simulink model "xplane2matlab"  (R2016a)
settings: Solver=ode45  StartTime=0.0  StopTime=inf  RelTol=1e-3
libraries: xpcutilitieslib x2, xpcobsoletelib x2, instrumentlib x2
settings Model: Creator=IEE12  LastModifiedBy=Marcelo
settings DataIOCC: LimitDataPoints=on  SaveFormat=Array
settings DebuggingCC: UnderspecifiedInitializationDetection=Classic  MergeDetectMultiDrivingBlocksExec=none  SolverPrmCheckMsg=warning  StateNameClashWarn=warning
settings HardwareCC: ProdBitPerPointer=32  ProdLargestAtomicFloat=None  ProdIntDivRoundTo=Undefined  ProdEndianess=Unspecified  ProdWordSize=32  ProdHWDeviceType=32-bit Generic
settings ModelReferenceCC: PropagateSignalLabelsOutOfModel=off
settings ConfigComp: CovModelRefEnable=Off

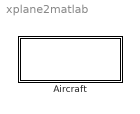
== system xplane2matlab ==
  Aircraft : Subsystem

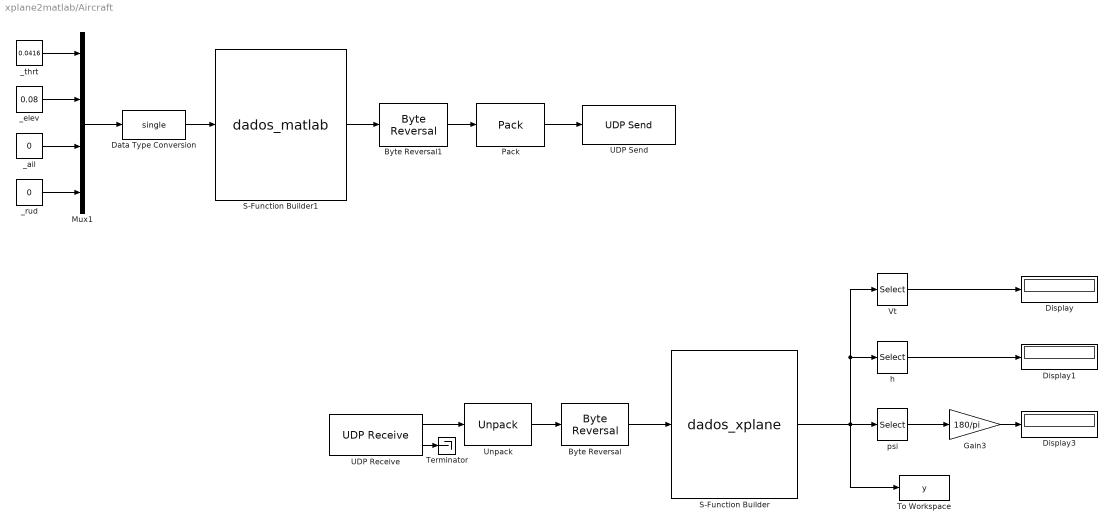
== system xplane2matlab/Aircraft ==
  Byte Reversal : xpcutilitieslib/Byte Reversal   numInp=1
  Byte Reversal1 : xpcutilitieslib/Byte Reversal   numInp=1
  Data Type Conversion : DataTypeConversion  OutDataTypeStr=single
  Display : Display
  Display1 : Display
  Display3 : Display
  Gain3 : Gain  Gain=180/pi
  Mux1 : Mux
  Pack : xpcobsoletelib/Utilities/Pack   datatypes={'uint8'}  byteAlign=1
  S-Function Builder : S-Function  InitFcn=try, set_param(gcb,'FunctionName','dados_xplane'), end  FunctionName=dados_xplane  SFunctionModules=dados_xplane_wrapper  SFunctionDeploymentMode=off  EnableBusSupport=off  mask(S-Function Builder){}
      mask help: Simulink:masks:SFunctionBuilder_MD
      mask init:
      | val = [[.9  0.75 0.75 1 1 .9 .9 1]',[1 1 0.75 0.75 .9 .9 1 .9]'];try , sys = get_param(gcb,'SfunBuilderFcnName');if isempty(sys), sys = get_param(gcb,'FunctionName'); end,catch, sys = get_param(gcb,'FunctionName'); end
      settings: CopyFcn=set_param(gcbh,'LinkStatus','none')  PreSaveFcn=try, set_param(gcb,'FunctionName','dados_xplane'), end  OpenFcn=sfunctionwizard(gcbh)
      mask Display: plot(val(:,1),val(:,2)),disp(sys), port_label('input',1,'Pkt'), port_label('output',1,'y')
  S-Function Builder1 : S-Function  InitFcn=try, set_param(gcb,'FunctionName','dados_matlab'), end  FunctionName=dados_matlab  SFunctionModules=dados_matlab_wrapper crc  SFunctionDeploymentMode=off  EnableBusSupport=off  mask(S-Function Builder){}
      mask help: Simulink:masks:SFunctionBuilder_MD
      mask init: same as xplane2matlab/Aircraft/S-Function Builder
      settings: CopyFcn=set_param(gcbh,'LinkStatus','none')  PreSaveFcn=try, set_param(gcb,'FunctionName','dados_matlab'), end  OpenFcn=sfunctionwizard(gcbh)
      mask Display: plot(val(:,1),val(:,2)),disp(sys), port_label('input',1,'u'), port_label('output',1,'Pkt')
  Terminator : Terminator
  To Workspace : ToWorkspace  VariableName=y  SaveFormat=Timeseries  SampleTime=-1
  UDP Receive : instrumentlib/UDP Receive  Host=127.0.0.1  Port=45004  LocalPort=45001  DataSize=77  EnableBlockingMode=off  Timeout=10  SampleTime=0.02  DataType=uint8  ByteOrder=BigEndian
  UDP Send : instrumentlib/UDP Send  Host=127.0.0.1  Port=45004  LocalPort=45001  EnableBlockingMode=on  ByteOrder=BigEndian
  Unpack : xpcobsoletelib/Utilities/Unpack   dimensions={[1 77]}  datatypes={'uint8'}  byteAlign=1
  Vt : Selector  InputPortWidth=12  IndexOptions=Index vector (dialog)  Indices=[1]  OutputSizes=1
  _ail : Constant  Value=0
  _elev : Constant  Value=0.08
  _rud : Constant  Value=0
  _thrt : Constant  Value=0.0416
  h : Selector  InputPortWidth=12  IndexOptions=Index vector (dialog)  Indices=[12]  OutputSizes=1
  psi : Selector  InputPortWidth=12  IndexOptions=Index vector (dialog)  Indices=[9]  OutputSizes=1
  wires:
  UDP Receive/2 -> Terminator/1
  UDP Receive/1 -> Unpack/1
  Unpack/1 -> Byte Reversal/1
  Byte Reversal/1 -> S-Function Builder/1
  Byte Reversal1/1 -> Pack/1
  S-Function Builder1/1 -> Byte Reversal1/1
  Pack/1 -> UDP Send/1
  Mux1/1 -> Data Type Conversion/1
  _elev/1 -> Mux1/2
  _rud/1 -> Mux1/4
  _thrt/1 -> Mux1/1
  _ail/1 -> Mux1/3
  Data Type Conversion/1 -> S-Function Builder1/1
  psi/1 -> Gain3/1
  S-Function Builder/1 -> To Workspace/1, Vt/1, h/1, psi/1
  Vt/1 -> Display/1
  h/1 -> Display1/1
  Gain3/1 -> Display3/1
